simulink model "testing_mfunction"  (R2018b)
settings: Solver=VariableStepAuto  StartTime=0.0  StopTime=10.0  RelTol=1e-3
settings Model: Creator=bradyplanden  LastModifiedBy=bradyplanden

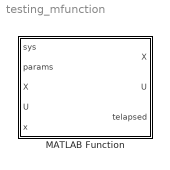
== system testing_mfunction ==
  MATLAB Function : MATLAB Function  TreatAsAtomicUnit=on

== matlab function testing_mfunction/MATLAB Function ==
  data: sys input; X output; params input; X input; U input; x input; U output; telapsed output
function [X,U,telapsed] = fcn(sys,params,X,U,x)

[X,U,telapsed] = fmpc_step(sys,params,X,U,x);
